simulink model "simulacionPlantaControlada"
settings: Solver=ode45  StartTime=0.0  StopTime=3  RelTol=1e-3
values from neighbouring files (symbols this model uses):
  a = [0  1  0; 0  0  1; -792900  -79150  -14.01]    [workspace.mat]
  adis = [0.914511514614  0.00121885851927  2.32580878052e-05; -18.4413378208  -0.92636613517  0.000893012709119; -708.069777061  -89.1232937476  -0.938877243225]    [workspace.mat]
  b = [7.711 -167.9 63100]    [workspace.mat]
  bdis = [0.0778470295061 0.60373728431 237.584820105]    [workspace.mat]
  c = [1 0 0]    [workspace.mat]
  cdis = [1 0 0]    [workspace.mat]
  h = [15.99 -79074.0199 -949681.481201]    [workspace.mat]
  hdis = [-3.66524411789 2900.58437447 278392.237488]    [workspace.mat]
  ki = -23.6307990829    [workspace.mat]
  kidis = -0.214176857697    [workspace.mat]
  kp = [2.35890748821 0.000417540035136 2.98030004827e-05]    [workspace.mat]
  kpdis = [2.2447842013 0.000170881301687 2.70063447362e-05]    [workspace.mat]
  tm = 0.01    [workspace.mat]
settings Model: Creator=automatica  LastModifiedBy=automatica
settings DataIOCC: LimitDataPoints=on  SaveFormat=Array  SignalLoggingSaveFormat=ModelDataLogs  ReturnWorkspaceOutputs=off
settings OptimizationCC: ExpressionDepthLimit=2147483647  LifeSpan=inf  SimCompilerOptimization=Off
settings DebuggingCC: UnderspecifiedInitializationDetection=Classic  MergeDetectMultiDrivingBlocksExec=none  SolverPrmCheckMsg=warning  MultiTaskDSMMsg=warning  MultiTaskCondExecSysMsg=none  FcnCallInpInsideContextMsg=Enable All  FrameProcessingCompatibilityMsg=warning  StateNameClashWarn=warning  StrictBusMsg=None  SFUnexpectedBacktrackingDiag=warning  SFNoUnconditionalDefaultTransitionDiag=warning
settings HardwareCC: ProdBitPerPointer=32  ProdLargestAtomicFloat=None  ProdIntDivRoundTo=Undefined  ProdEndianess=Unspecified  ProdWordSize=32  ProdHWDeviceType=32-bit Generic
settings ModelReferenceCC: PropagateSignalLabelsOutOfModel=off
settings SFSimCC: SimUseLocalCustomCode=off
settings RTWCC: RTWUseLocalCustomCode=off  IncludeERTFirstTime=on  RTWCompilerOptimization=Off
settings CodeAppCC: CustomSymbolStrType=$N$R$M
settings GRTTargetCC: CodeReplacementLibrary=ANSI_C  GeneratePreprocessorConditionals=Disable all  CPPClassGenCompliant=off

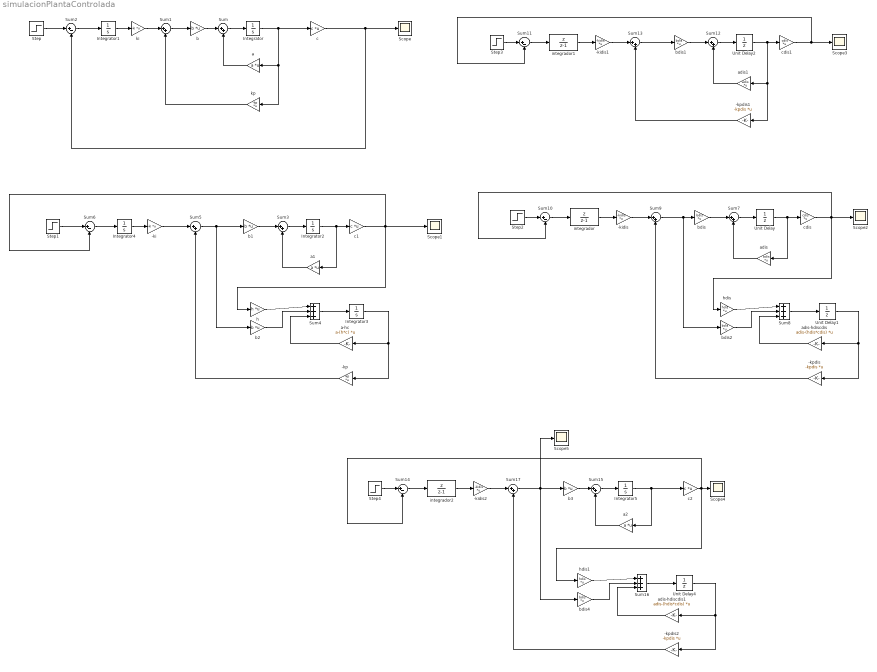
== system simulacionPlantaControlada ==
  -ki : Gain  Gain=-ki  Multiplication=Matrix(K*u) (u vector)
  -kidis : Gain  Gain=-kidis  Multiplication=Matrix(K*u) (u vector)  SampleTime=tm
  -kidis1 : Gain  Gain=-kidis  Multiplication=Matrix(K*u) (u vector)  SampleTime=tm
  -kidis2 : Gain  Gain=-kidis  Multiplication=Matrix(K*u) (u vector)  SampleTime=tm
  -kp : Gain  Gain=-kp  Multiplication=Matrix(K*u) (u vector)
  -kpdis : Gain  Gain=-kpdis  Multiplication=Matrix(K*u) (u vector)  SampleTime=tm
  -kpdis1 : Gain  Gain=-kpdis  Multiplication=Matrix(K*u) (u vector)  SampleTime=tm
  -kpdis2 : Gain  Gain=-kpdis  Multiplication=Matrix(K*u) (u vector)  SampleTime=tm
  Integrator{,1..5} (6 alike) : Integrator
  Scope{,1..5} (6 alike) : Scope
      Scope2 settings: SaveName=ScopeData2
      Scope3 settings: SaveName=ScopeData3
      Scope4 settings: SaveName=ScopeData4
      Scope5 settings: SaveName=ScopeData5
  Step : Step  Time=0  After=5  SampleTime=0
  Step1 : Step  Time=0  After=5  SampleTime=0
  Step2 : Step  Time=0  After=5  SampleTime=tm
  Step3 : Step  Time=0  After=5  SampleTime=tm
  Step4 : Step  Time=0  After=5  SampleTime=tm
  Sum{,1,3,5,15} (5 alike) : Sum  Inputs=|++
  Sum10 : Sum  Inputs=|+-  SampleTime=tm
  Sum11 : Sum  Inputs=|+-  SampleTime=tm
  Sum{7,9,12..13,17} (5 alike) : Sum  Inputs=|++  SampleTime=tm
  Sum14 : Sum  Inputs=|+-  SampleTime=tm
  Sum16 : Sum  Inputs=|+++  SampleTime=tm
  Sum2 : Sum  Inputs=|+-
  Sum4 : Sum  Inputs=|+++
  Sum6 : Sum  Inputs=|+-
  Sum8 : Sum  Inputs=|+++  SampleTime=tm
  Unit Delay{,1..2,4} (4 alike) : UnitDelay  SampleTime=tm
  a : Gain  Gain=a  Multiplication=Matrix(K*u) (u vector)
  a-hc : Gain  Gain=a-(h*c)  Multiplication=Matrix(K*u) (u vector)
  a1 : Gain  Gain=a  Multiplication=Matrix(K*u) (u vector)
  a2 : Gain  Gain=a  Multiplication=Matrix(K*u) (u vector)
  adis : Gain  Gain=adis  Multiplication=Matrix(K*u) (u vector)  SampleTime=tm
  adis-hdiscdis : Gain  Gain=adis-(hdis*cdis)  Multiplication=Matrix(K*u) (u vector)  SampleTime=tm
  adis-hdiscdis1 : Gain  Gain=adis-(hdis*cdis)  Multiplication=Matrix(K*u) (u vector)  SampleTime=tm
  adis1 : Gain  Gain=adis  Multiplication=Matrix(K*u) (u vector)  SampleTime=tm
  b{,1..3} (4 alike) : Gain  Gain=b  Multiplication=Matrix(K*u) (u vector)
  bdis{,1..2,4} (4 alike) : Gain  Gain=bdis  Multiplication=Matrix(K*u) (u vector)  SampleTime=tm
  c : Gain  Gain=c  Multiplication=Matrix(K*u) (u vector)
  c1 : Gain  Gain=c  Multiplication=Matrix(K*u) (u vector)
  c2 : Gain  Gain=c  Multiplication=Matrix(K*u) (u vector)
  cdis : Gain  Gain=cdis  Multiplication=Matrix(K*u) (u vector)  SampleTime=tm
  cdis1 : Gain  Gain=cdis  Multiplication=Matrix(K*u) (u vector)  SampleTime=tm
  h : Gain  Gain=h  Multiplication=Matrix(K*u) (u vector)
  hdis : Gain  Gain=hdis  Multiplication=Matrix(K*u) (u vector)  SampleTime=tm
  hdis1 : Gain  Gain=hdis  Multiplication=Matrix(K*u) (u vector)  SampleTime=tm
  integrador : DiscreteTransferFcn  Numerator=[1 0]  Denominator=[1 -1]  SampleTime=tm
  integrador1 : DiscreteTransferFcn  Numerator=[1 0]  Denominator=[1 -1]  SampleTime=tm
  integrador2 : DiscreteTransferFcn  Numerator=[1 0]  Denominator=[1 -1]  SampleTime=tm
  ki : Gain  Gain=-ki  Multiplication=Matrix(K*u) (u vector)
  kp : Gain  Gain=-kp  Multiplication=Matrix(K*u) (u vector)
  wires:
  b/1 -> Sum/1
  Sum/1 -> Integrator/1
  Integrator/1 -> c/1, a/1, kp/1
  a/1 -> Sum/2
  kp/1 -> Sum1/2
  ki/1 -> Sum1/1
  Sum1/1 -> b/1
  Integrator1/1 -> ki/1
  Step/1 -> Sum2/1
  Sum2/1 -> Integrator1/1
  c/1 -> Sum2/2, Scope/1
  b1/1 -> Sum3/1
  Sum3/1 -> Integrator2/1
  Integrator2/1 -> a1/1, c1/1
  a1/1 -> Sum3/2
  h/1 -> Sum4/1
  b2/1 -> Sum4/2
  Sum4/1 -> Integrator3/1
  Integrator3/1 -> -kp/1, a-hc/1
  a-hc/1 -> Sum4/3
  Sum5/1 -> b2/1, b1/1
  -kp/1 -> Sum5/2
  -ki/1 -> Sum5/1
  Integrator4/1 -> -ki/1
  Sum6/1 -> Integrator4/1
  Step1/1 -> Sum6/1
  c1/1 -> h/1, Sum6/2, Scope1/1
  bdis/1 -> Sum7/1
  Sum7/1 -> Unit Delay/1
  Unit Delay/1 -> adis/1, cdis/1
  adis/1 -> Sum7/2
  hdis/1 -> Sum8/1
  bdis2/1 -> Sum8/2
  Sum8/1 -> Unit Delay1/1
  Unit Delay1/1 -> -kpdis/1, adis-hdiscdis/1
  adis-hdiscdis/1 -> Sum8/3
  Sum9/1 -> bdis2/1, bdis/1
  -kidis/1 -> Sum9/1
  integrador/1 -> -kidis/1
  Sum10/1 -> integrador/1
  Step2/1 -> Sum10/1
  -kpdis/1 -> Sum9/2
  cdis/1 -> Sum10/2, hdis/1, Scope2/1
  bdis1/1 -> Sum12/1
  Sum12/1 -> Unit Delay2/1
  Unit Delay2/1 -> -kpdis1/1, adis1/1, cdis1/1
  adis1/1 -> Sum12/2
  Sum13/1 -> bdis1/1
  -kidis1/1 -> Sum13/1
  integrador1/1 -> -kidis1/1
  Sum11/1 -> integrador1/1
  Step3/1 -> Sum11/1
  cdis1/1 -> Sum11/2, Scope3/1
  -kpdis1/1 -> Sum13/2
  hdis1/1 -> Sum16/1
  bdis4/1 -> Sum16/2
  Sum16/1 -> Unit Delay4/1
  Unit Delay4/1 -> -kpdis2/1, adis-hdiscdis1/1
  adis-hdiscdis1/1 -> Sum16/3
  Sum17/1 -> bdis4/1, b3/1, Scope5/1
  -kidis2/1 -> Sum17/1
  integrador2/1 -> -kidis2/1
  Sum14/1 -> integrador2/1
  Step4/1 -> Sum14/1
  -kpdis2/1 -> Sum17/2
  b3/1 -> Sum15/1
  Sum15/1 -> Integrator5/1
  Integrator5/1 -> c2/1, a2/1
  a2/1 -> Sum15/2
  c2/1 -> Scope4/1, Sum14/2, hdis1/1
